simulink model "qless_forgetting_factor_16x16"  (R2021a)
settings: Solver=FixedStepDiscrete  StartTime=0.0  StopTime=stoptime*inf  RelTol=1e-3
InitFcn:
  | qless_init_16chan_fi
undefined symbols (not defined in the file): fc, numArrayElements, physconst, srcAngles, sv, Ts
libraries: hdlsllib x137, commfilt2 x4, commrfcorlib x3, commsync2 x3, commrflib2 x2, commrandsrc3 x2, phasedtxrxlib x2, commdigbbndcpm2 x1, simulink x1, embreciprocals x1, commdigbbndpm3 x1
(part 19 of 22)

== matlab function qless_forgetting_factor_16x16/MVDR_QLess_HDL/Complex Partial-Systolic Matrix Solve Using Q-less QR Decomposition with Forgetting Factor Manually Tiled n=16/Complex Partial-Systolic Q-less QR with Forgetting Factor/Complex Partial-Systolic Q-less QR with Forgetting Factor Manually tiled/Shorten by one3 ==
  data: u input; y output
function y = shorten_by_1(u)
    y = u(2:end);
end

== matlab function qless_forgetting_factor_16x16/MVDR_QLess_HDL/Complex Partial-Systolic Matrix Solve Using Q-less QR Decomposition with Forgetting Factor Manually Tiled n=16/Complex Partial-Systolic Q-less QR with Forgetting Factor/Complex Partial-Systolic Q-less QR with Forgetting Factor Manually tiled/Shorten by one4 ==
  data: u input; y output
function y = shorten_by_1(u)
    y = u(2:end);
end

== matlab function qless_forgetting_factor_16x16/MVDR_QLess_HDL/Complex Partial-Systolic Matrix Solve Using Q-less QR Decomposition with Forgetting Factor Manually Tiled n=16/Complex Partial-Systolic Q-less QR with Forgetting Factor/Complex Partial-Systolic Q-less QR with Forgetting Factor Manually tiled/Shorten by one5 ==
  data: u input; y output
function y = shorten_by_1(u)
    y = u(2:end);
end

== matlab function qless_forgetting_factor_16x16/MVDR_QLess_HDL/Complex Partial-Systolic Matrix Solve Using Q-less QR Decomposition with Forgetting Factor Manually Tiled n=16/Complex Partial-Systolic Q-less QR with Forgetting Factor/Complex Partial-Systolic Q-less QR with Forgetting Factor Manually tiled/Shorten by one6 ==
  data: u input; y output
function y = shorten_by_1(u)
    y = u(2:end);
end

== matlab function qless_forgetting_factor_16x16/MVDR_QLess_HDL/Complex Partial-Systolic Matrix Solve Using Q-less QR Decomposition with Forgetting Factor Manually Tiled n=16/Complex Partial-Systolic Q-less QR with Forgetting Factor/Complex Partial-Systolic Q-less QR with Forgetting Factor Manually tiled/Shorten by one7 ==
  data: u input; y output
function y = shorten_by_1(u)
    y = u(2:end);
end

== matlab function qless_forgetting_factor_16x16/MVDR_QLess_HDL/Complex Partial-Systolic Matrix Solve Using Q-less QR Decomposition with Forgetting Factor Manually Tiled n=16/Complex Partial-Systolic Q-less QR with Forgetting Factor/Complex Partial-Systolic Q-less QR with Forgetting Factor Manually tiled/Shorten by one8 ==
  data: u input; y output
function y = shorten_by_1(u)
    y = u(2:end);
end

== matlab function qless_forgetting_factor_16x16/MVDR_QLess_HDL/Complex Partial-Systolic Matrix Solve Using Q-less QR Decomposition with Forgetting Factor Manually Tiled n=16/Complex Partial-Systolic Q-less QR with Forgetting Factor/Complex Partial-Systolic Q-less QR with Forgetting Factor Manually tiled/Shorten by one10 ==
  data: u input; y output
function y = shorten_by_1(u)
    y = u(2:end);
end

== matlab function qless_forgetting_factor_16x16/MVDR_QLess_HDL/Complex Partial-Systolic Matrix Solve Using Q-less QR Decomposition with Forgetting Factor Manually Tiled n=16/Complex Partial-Systolic Q-less QR with Forgetting Factor/Complex Partial-Systolic Q-less QR with Forgetting Factor Manually tiled/Shorten by one11 ==
  data: u input; y output
function y = shorten_by_1(u)
    y = u(2:end);
end

== matlab function qless_forgetting_factor_16x16/MVDR_QLess_HDL/Complex Partial-Systolic Matrix Solve Using Q-less QR Decomposition with Forgetting Factor Manually Tiled n=16/Complex Partial-Systolic Q-less QR with Forgetting Factor/Complex Partial-Systolic Q-less QR with Forgetting Factor Manually tiled/Shorten by one12 ==
  data: u input; y output
function y = shorten_by_1(u)
    y = u(2:end);
end

== matlab function qless_forgetting_factor_16x16/MVDR_QLess_HDL/Complex Partial-Systolic Matrix Solve Using Q-less QR Decomposition with Forgetting Factor Manually Tiled n=16/Complex Partial-Systolic Q-less QR with Forgetting Factor/Complex Partial-Systolic Q-less QR with Forgetting Factor Manually tiled/Shorten by one13 ==
  data: u input; y output
function y = shorten_by_1(u)
    y = u(2:end);
end

== matlab function qless_forgetting_factor_16x16/MVDR_QLess_HDL/Complex Partial-Systolic Matrix Solve Using Q-less QR Decomposition with Forgetting Factor Manually Tiled n=16/Complex Partial-Systolic Q-less QR with Forgetting Factor/Complex Partial-Systolic Q-less QR with Forgetting Factor Manually tiled/Complex Partial-Systolic Q-less QR Decomposition with Forgetting Factor Section Constant pivot1/Complex Partial-Systolic Q-less QR Row Rotations/Inverse CORDIC Gain1/MATLAB Function ==
  data: u input; y output
function y = inverseCORDICGain(u)
    %inverseCORDICGain Multiply by the inverse of the CORDIC gain constant
    %   Y = inverseCORDICGain(U) multiplies input U by the inverse CORDIC
    %   gain constant.  The data type of output Y is the same as the data
    %   type of input U.  This data type will never overflow because the
    %   inverse CORDIC gain constant quickly converges to around 0.60725 as
    %   a function of the word length of the input.
    F = fixed.fimathLike(u);
    [~, Kn] = fixed.cordicConstants(u);
    y = setfimath(u,F) * Kn;
end

== matlab function qless_forgetting_factor_16x16/MVDR_QLess_HDL/Complex Partial-Systolic Matrix Solve Using Q-less QR Decomposition with Forgetting Factor Manually Tiled n=16/Complex Partial-Systolic Q-less QR with Forgetting Factor/Complex Partial-Systolic Q-less QR with Forgetting Factor Manually tiled/Complex Partial-Systolic Q-less QR Decomposition with Forgetting Factor Section Constant pivot1/Complex Partial-Systolic Q-less QR Row Rotations/Inverse CORDIC Gain4/MATLAB Function ==
  data: u input; y output
function y = inverseCORDICGain(u)
    %inverseCORDICGain Multiply by the inverse of the CORDIC gain constant
    %   Y = inverseCORDICGain(U) multiplies input U by the inverse CORDIC
    %   gain constant.  The data type of output Y is the same as the data
    %   type of input U.  This data type will never overflow because the
    %   inverse CORDIC gain constant quickly converges to around 0.60725 as
    %   a function of the word length of the input.
    F = fixed.fimathLike(u);
    [~, Kn] = fixed.cordicConstants(u);
    y = setfimath(u,F) * Kn;
end

== matlab function qless_forgetting_factor_16x16/MVDR_QLess_HDL/Complex Partial-Systolic Matrix Solve Using Q-less QR Decomposition with Forgetting Factor Manually Tiled n=16/Complex Partial-Systolic Q-less QR with Forgetting Factor/Complex Partial-Systolic Q-less QR with Forgetting Factor Manually tiled/Complex Partial-Systolic Q-less QR Decomposition with Forgetting Factor Section Constant pivot1/Complex Partial-Systolic Q-less QR Row Rotations/Q-less QR Rotate First Element To Real1/Q-less QR Real Row Rotations/Inverse CORDIC Gain/MATLAB Function ==
  data: u input; y output
function y = inverseCORDICGain(u)
    %inverseCORDICGain Multiply by the inverse of the CORDIC gain constant
    %   Y = inverseCORDICGain(U) multiplies input U by the inverse CORDIC
    %   gain constant.  The data type of output Y is the same as the data
    %   type of input U.  This data type will never overflow because the
    %   inverse CORDIC gain constant quickly converges to around 0.60725 as
    %   a function of the word length of the input.
    F = fixed.fimathLike(u);
    [~, Kn] = fixed.cordicConstants(u);
    y = setfimath(u,F) * Kn;
end

== matlab function qless_forgetting_factor_16x16/MVDR_QLess_HDL/Complex Partial-Systolic Matrix Solve Using Q-less QR Decomposition with Forgetting Factor Manually Tiled n=16/Complex Partial-Systolic Q-less QR with Forgetting Factor/Complex Partial-Systolic Q-less QR with Forgetting Factor Manually tiled/Complex Partial-Systolic Q-less QR Decomposition with Forgetting Factor Section Constant pivot1/Complex Partial-Systolic Q-less QR Row Rotations/Q-less QR Rotate First Element To Real1/Q-less QR Real Row Rotations/Inverse CORDIC Gain1/MATLAB Function ==
  data: u input; y output
function y = inverseCORDICGain(u)
    %inverseCORDICGain Multiply by the inverse of the CORDIC gain constant
    %   Y = inverseCORDICGain(U) multiplies input U by the inverse CORDIC
    %   gain constant.  The data type of output Y is the same as the data
    %   type of input U.  This data type will never overflow because the
    %   inverse CORDIC gain constant quickly converges to around 0.60725 as
    %   a function of the word length of the input.
    F = fixed.fimathLike(u);
    [~, Kn] = fixed.cordicConstants(u);
    y = setfimath(u,F) * Kn;
end

== matlab function qless_forgetting_factor_16x16/MVDR_QLess_HDL/Complex Partial-Systolic Matrix Solve Using Q-less QR Decomposition with Forgetting Factor Manually Tiled n=16/Complex Partial-Systolic Q-less QR with Forgetting Factor/Complex Partial-Systolic Q-less QR with Forgetting Factor Manually tiled/Complex Partial-Systolic Q-less QR Decomposition with Forgetting Factor Section Constant pivot1/Complex Partial-Systolic Q-less QR Row Rotations/Q-less QR Rotate First Element To Real1/Q-less QR Real Row Rotations/Q-less QR Real Indexed CORDIC Row Rotation/CORDIC QR Kernel ==
  settings: fimath=hdlfimath
  data: xIn input size=n; yIn input size=n; validIn input; restart input; xOut output size=n; yOut output size=n; n parameter; validOut output boolean; ready output; pivot parameter size=1
function [xOut, yOut, validOut, ready] = cordic_qr_row_rotation(...
                                                xIn, yIn,...
                                                validIn,...
                                                restart,...
                                                n, pivot)... 
    %CORDIC_QR_ROW_ROTATION performs one CORDIC Givens rotation
    % [XOUT, YOUT] = CORDIC_QR_ROW_ROTATION(...
    %                                       XREG,YREG,...
    %                                       XIN,YIN,...
    %                                       PIVOT,...
    %                                       STILLITERATING, ITERATION)
    % performs one iteration of the CORDIC Givens rotation according to
    % the formula below.
    %
    % if real(y(column)) < 0
    %       xOut = x - y/2^iteration
    %       yOut = y + x/2^iteration
    %   else
    %       xOut = x + y/2^iteration
    %       yOut = y - x/2^iteration
    % end
    %
    % The values for X, Y, are taken from XIN, YIN, on the first iteration, 
    % and XREG, YREG on succeeding iterations.
    
    %   Copyright 2018 The MathWorks, Inc.
    
    %#codegen
    
    % Initialize variables to set datatypes
    
    persistent xReg yReg count readyReg
    
    
    
    fixed.emblib.internal.cordicRowRotations.checkValidDatatypes(xIn, yIn,'x','y', 'cordic_qr_row_rotation');
    T = fixed.emblib.internal.cordicRowRotations.getTypesTable(xIn,xIn);
    maxNIters = coder.const(fixed.emblib.internal.cordicRowRotations.getMaxNIters(xIn));
    
    if isempty(xReg)
       xReg = zeros(n,1,'like',T.x);
       yReg = zeros(n,1,'like',T.y);
       count = cast(0,'like',T.count);
       readyReg = true;
    end
    
    if validIn
        iteration = cast(0,'like',count);
        x = cast(xIn,'like',T.x);
        y = cast(yIn,'like',T.y);
    else
        iteration = count;
        x = xReg;
        y = yReg;
    end
    
    
    [xNext, yNext] = cordicQlessQRRowRotation(x, y, iteration, pivot, T);
    incrCounter =  (validIn && readyReg) || (iteration > 0 && iteration < maxNIters);
    if restart || ~incrCounter
        iterationNext = cast(0,'like',T.count);
    else
        iterationNext = cast(iteration + 1,'like',T.count);
    end
    
    if restart || (iteration == maxNIters - 1)
        readyNext = true;
    elseif validIn && ~readyReg
        readyNext = false;
    else
        readyNext = readyReg;
    end
        
        
    % Set the output
    xOut = xNext;
    yOut = yNext;
    if iteration == maxNIters - 1
        validOut = true;
        % Set the registers to zero to prevent overflows being reported on
        % CORDIC iterations over invalid data.
        xReg(:) = 0;
        yReg(:) = 0;
    else
        validOut = false;
        % Still iterating, so update the registers with next values.
        xReg(:) = xNext;
        yReg(:) = yNext;
    end
    ready = readyNext;
    % Update the registers
    count(:) = iterationNext;
    readyReg(:) = readyNext;
    
    
end

function [xOut, yOut] = cordicQlessQRRowRotation(x, y,...
        iteration, pivot, T)
%cordicQlessQRRowRotation One iteration of the Q-less QR CORDIC kernel
%   [XOUT, YOUT] = cordicQlessQRRowRotation(X,Y,...
%                                      ITERATION, PIVOT, T)
%   performs a single CORDIC Givens rotation according to the
%   formula below
%
%   if real(y(pivot)) < 0
%       xOut = x - y/2^iteration
%       yOut = y + x/2^iteration
%   else
%       xOut = x + y/2^iteration
%       yOut = y - x/2^iteration
%   end

    coder.inline('always');
    
    % Initialize output variables
    xOut = cast(x,'like',T.x);
    yOut = cast(y,'like',T.y);
    % Right shift the inputs for CORDIC rotations.
    x1 = zeros(size(x),'like',x);
    y1 = zeros(size(y),'like',y);
    coder.unroll
    for k = pivot:length(x)
        x1(k) = bitsra(x(k), iteration);
        y1(k) = bitsra(y(k), iteration);
    end
    if real(y(pivot)) < 0
        % Counter-clockwise rotation
        coder.unroll
        for k = pivot:length(x)
            xOut(k) = x(k) - y1(k);
            yOut(k) = y(k) + x1(k);
        end
    else
        % Clockwise rotation
        coder.unroll
        for k = pivot:length(x)
            xOut(k) = x(k) + y1(k);
            yOut(k) = y(k) - x1(k);
        end
    end
end

== matlab function qless_forgetting_factor_16x16/MVDR_QLess_HDL/Complex Partial-Systolic Matrix Solve Using Q-less QR Decomposition with Forgetting Factor Manually Tiled n=16/Complex Partial-Systolic Q-less QR with Forgetting Factor/Complex Partial-Systolic Q-less QR with Forgetting Factor Manually tiled/Complex Partial-Systolic Q-less QR Decomposition with Forgetting Factor Section Constant pivot1/Complex Partial-Systolic Q-less QR Row Rotations/Q-less QR Rotate First Element To Real1/Q-less QR Real Row Rotations/Set Element To Zero/Set Element To Zero ==
  settings: fimath=hdlfimath
  data: u input size=[1 n]; y output size=[1 n]; n parameter; pivot parameter size=1
function y = set_element_equal_to_zero(u, n, pivot)
    % SET_ELEMENT_EQUAL_TO_ZERO Zeros an element for a row-vector.
    %   Y = SET_ELEMENT_EQUAL_TO_ZERO(U, PIVOT) sets an element
    %   (specified by PIVOT) of the row-vector U to zero.

    %   Copyright 2018 The MathWorks, Inc.

    %# codegen
    assert(isequal(size(u),[1,n]));
    y = u;
    if pivot > 0 && pivot <= n
        y(pivot) = 0;
    end
end

== matlab function qless_forgetting_factor_16x16/MVDR_QLess_HDL/Complex Partial-Systolic Matrix Solve Using Q-less QR Decomposition with Forgetting Factor Manually Tiled n=16/Complex Partial-Systolic Q-less QR with Forgetting Factor/Complex Partial-Systolic Q-less QR with Forgetting Factor Manually tiled/Shorten by one14 ==
  data: u input; y output
function y = shorten_by_1(u)
    y = u(2:end);
end

== matlab function qless_forgetting_factor_16x16/MVDR_QLess_HDL/Complex Partial-Systolic Matrix Solve Using Q-less QR Decomposition with Forgetting Factor Manually Tiled n=16/Complex Partial-Systolic Q-less QR with Forgetting Factor/Complex Partial-Systolic Q-less QR with Forgetting Factor Manually tiled/Complex Partial-Systolic Q-less QR Decomposition with Forgetting Factor Section Constant pivot1/Complex Partial-Systolic Q-less QR Row Rotations/Set Element To Zero1/Set Element To Zero ==
  settings: fimath=hdlfimath
  data: u input size=[1 n]; y output size=[1 n]; n parameter; pivot parameter size=1
function y = set_element_equal_to_zero(u, n, pivot)
    % SET_ELEMENT_EQUAL_TO_ZERO Zeros an element for a row-vector.
    %   Y = SET_ELEMENT_EQUAL_TO_ZERO(U, PIVOT) sets an element
    %   (specified by PIVOT) of the row-vector U to zero.

    %   Copyright 2018 The MathWorks, Inc.

    %# codegen
    assert(isequal(size(u),[1,n]));
    y = u;
    if pivot > 0 && pivot <= n
        y(pivot) = 0;
    end
end

== matlab function qless_forgetting_factor_16x16/MVDR_QLess_HDL/Complex Partial-Systolic Matrix Solve Using Q-less QR Decomposition with Forgetting Factor Manually Tiled n=16/Complex Partial-Systolic Q-less QR with Forgetting Factor/Complex Partial-Systolic Q-less QR with Forgetting Factor Manually tiled/Complex Partial-Systolic Q-less QR Decomposition with Forgetting Factor Section Constant pivot1/Partial-Systolic Q-less QR with Forgetting Factor Memory Controller/MATLAB Function ==
  data: xIn input; xOut output; aIn input; validIn input size=1; validRowRotationInput input size=1; restart input size=1; yOut output; processRowRotations output size=1; validOut output size=1; ready output size=1; n parameter size=1
function [...
        xOut,...
        yOut,...
        processRowRotations,...
        validOut,...
        ready...
        ] = ...
        partialSystolicQlessQRMemoryControllerForgettingFactorMATLAB(...
        xIn,...
        aIn,...
        validIn,...
        validRowRotationInput,...
        restart, ...
        n)
    
    % Persistent states
    persistent mState
    persistent mRow
    persistent mR
    
    if isempty(mState)
        mState = uint8(0);
        mRow = uint16(1);
        mR = zeros(1,n,'like',aIn);
    end
    
    [...
        xOut,...
        yOut,...
        processRowRotations,...
        validOut,...
        ready,...
        mState,...
        mRow,...
        mR...
        ] = ...
        partialSystolicQlessQRMemoryControllerForgettingFactor(...
        xIn,...
        aIn,...
        validIn,...
        validRowRotationInput,...
        restart, ...
        n,...
        mState,...
        mRow,...
        mR);
end

function [...
        xOut,...
        yOut,...
        processRowRotations,...
        validOut,...
        ready,...
        mState,...
        mRowIndex,...
        mRow...
        ] = ...
        partialSystolicQlessQRMemoryControllerForgettingFactor(...
        xIn,...
        aIn,...
        validIn,...
        validRowRotationInput,...
        restart, ...
        n,...
        mState,...
        mRowIndex,...
        mRow)
    %partialSystolicQlessQRMemoryControllerForgettingFactor
    
    % Copyright 2020 The MathWorks, Inc.
    %#codegen
    
    % State names
    NEWMATRIX = uint8(0);
    GETROW = uint8(1);
    PROCESSPIVOT = uint8(2);
    OUTPUTROW = uint8(3);
    
    % Get states
    state = mState;
    row = mRowIndex;
    
    if restart
        state = NEWMATRIX;
    end
    
    % Default outputs.  States change them as needed.
    xOut = mRow;
    yOut = aIn;
    processRowRotations = false;
    validOut = false;
    ready = false;
    
    switch state
        case NEWMATRIX
            mRow(:) = 0;
            mRowIndex(:) = 1;
            mState(:) = GETROW;
            ready(:) = true;
        case GETROW
            if  validIn
                processRowRotations = true;
                mRowIndex(:) = row + 1;
                mState(:) = PROCESSPIVOT;
            else
                ready = true;
            end
        case PROCESSPIVOT
            if validRowRotationInput
                mRow(:) = xIn;
                if row > n
                    mState(:) = OUTPUTROW;
                else
                    mState(:) = GETROW;
                end
            end
        case OUTPUTROW
            validOut = true;
            mState(:) = GETROW;
    end
end

== matlab function qless_forgetting_factor_16x16/MVDR_QLess_HDL/Complex Partial-Systolic Matrix Solve Using Q-less QR Decomposition with Forgetting Factor Manually Tiled n=16/Complex Partial-Systolic Q-less QR with Forgetting Factor/Complex Partial-Systolic Q-less QR with Forgetting Factor Manually tiled/Shorten by one9 ==
  data: u input; y output
function y = shorten_by_1(u)
    y = u(2:end);
end

== matlab function qless_forgetting_factor_16x16/MVDR_QLess_HDL/Complex Partial-Systolic Matrix Solve Using Q-less QR Decomposition with Forgetting Factor Manually Tiled n=16/Complex Partial-Systolic Q-less QR with Forgetting Factor/Partial-Systolic Q-less QR with Forgetting Factor Output Memory Manager/Partial-Systolic Q-less QR Output Memory Manager1/Partial-Systolic Q-less QR Output State Machine ==
  data: writeEnable output; validIn input; restart input; m parameter size=1; n parameter size=1; validOut output
function [writeEnable,validOut] = qlessqrOutputMATLABFunctionBlock(validIn,restart,m,n)
    coder.internal.assert(m>=n,'fixed:emblib:MustBeTallAndSkinny','A');
    % State names
    NEWMATRIX = uint8(0);
    GETROW = uint8(1);
    persistent mWriteEnable;
    persistent mRowCounter
    persistent mPivot
    persistent mState
    persistent mValidOut
    if isempty(mWriteEnable)
        mWriteEnable = false(1,n);
        mRowCounter = uint32(0);
        mPivot = uint32(1);
        mState = GETROW;
        mValidOut = false;
    end
    writeEnable = mWriteEnable;
    validOut = mValidOut;
    
    state = mState;
    rowCounter = mRowCounter;
    pivot = mPivot;
    mValidOut = false;
    
    if restart
        state = NEWMATRIX;
    end
    mWriteEnable(:) = false;
    switch state
        case NEWMATRIX
            rowCounter(:) = 0;
            pivot(:) = 1;
            state(:) = GETROW;
        case GETROW
            if validIn(pivot)
                mWriteEnable(pivot) = true;
                pivot(:) = pivot + 1;
                if pivot > min(m,n)
                    rowCounter(:) = 1;
                    pivot(:) = 1;
                    mValidOut(:) = true;
                end
            end
        otherwise
    end
    
    mRowCounter(:) = rowCounter;
    mPivot(:) = pivot;
    mState(:) = state;
end

== matlab function qless_forgetting_factor_16x16/MVDR_QLess_HDL/Complex Partial-Systolic Matrix Solve Using Q-less QR Decomposition with Forgetting Factor Manually Tiled n=16/Complex Partial-Systolic Q-less QR with Forgetting Factor/Partial-Systolic Q-less QR with Forgetting Factor Output Memory Manager/Partial-Systolic Q-less QR Output Memory Manager1/Save Matrix Row/Enabled Delay ==
  data: dataIn input; dataOut output; writeEnable input
function dataOut = enabledDelay(dataIn,writeEnable)
    persistent mData
    if isempty(mData)
        mData = zeros(size(dataIn),'like',dataIn);
    end
    dataOut = mData;
    if writeEnable
        mData = dataIn;
    end
end

== matlab function qless_forgetting_factor_16x16/MVDR_QLess_HDL/Complex Partial-Systolic Matrix Solve Using Q-less QR Decomposition with Forgetting Factor Manually Tiled n=16/Complex Q-less QR Forward Backward Substitute/Complex Burst Back Substitute with Matrix Output1/Back substitute logic/Back substitute state machine ==
  settings: fimath=hdlfimath
  data: rowToSubtract1 output size=[1 p]; rowToSubtract2 output size=[1 p]; inverseElement input size=1; inverseShift input size=1; rIn input size=[1 n]; cIn input size=[1 p]; validIn input boolean size=1; start input boolean size=1; restart input boolean size=1; subtractedRow input size=[1 p]; addedRow input size=[1 p]; multipliedRow input size=[1 p]; finalMultipliedRow input size=[1 p]; rowToAdd1 output size=[1 p]; rowToAdd2 output size=[1 p]; rowToMultiply output size=[1 p]; rElement output size=1; finalRowToMultiply output size=[1 p]; reciprocal output size=1; shiftValue output size=1; xMatrix output size=[n p]; ready output boolean size=1; rowReady output boolean size=1; validOut output boolean size=1; n parameter size=1; p parameter size=1
function [rowToSubtract1,...
          rowToSubtract2,...
          rowToAdd1,...
          rowToAdd2,...
          rowToMultiply,...
          rElement,...
          finalRowToMultiply,...
          reciprocal,...
          shiftValue,...
          xMatrix,...
          ready,...
          rowReady,...
          validOut] = backsubStateMachine(inverseElement,...
                                          inverseShift,...
                                          rIn,...
                                          cIn,...
                                          validIn,...
                                          start,...
                                          restart,...
                                          subtractedRow,...
                                          addedRow,...
                                          multipliedRow,...
                                          finalMultipliedRow,...
                                          n,...
                                          p)
%backsubStateMachine Implements a state machine that manages the back
%substitute computation to compute the output matrix.
%
%   See also fixed.internal.matrixsolve.selectDiagonalElement.
%
%   Copyright 2019 The MathWorks, Inc.
%#codegen

%% INPUTS
% 'inverseElement' - The reciprocal of the diagonal element to be used
% later.
%
% 'inverseShift' - The reciprocal of the diagonal element is normalized,
% and needs to be denormalized later to yield the correct value.
%
% 'rIn' - A non-zero row of the R matrix from the QR decomposition.
%
% 'cIn' - A row of the Q'B matrix, where Q is obtained from the QR
% decomposition.
%
% 'validIn' - A boolean signal indicating that the data on the input lines
% is valid.
%
% 'start' - A boolean signal indicating that a new backsubstitute has
% begun; it thus indicates that new data should be expected.
%
% 'restart' - A boolean signal to reset the internal state of the block if
% necessary.
%
% 'subtractedRow' - The result of the subraction of the accumulated
% products of the non-diagonal elements of the supplied 'rIn' with the
% rows of the solution matrix, from 'cIn'.
%
% 'addedRow' - The accumulation of the products of the non-diagonal
% elements of the supplied 'rIn' with the rows of the solution matrix.
%
% 'multipliedRow' - The product of a non-diagonal element of the supplied
% 'rIn' with a row from the solution matrix.
%
% 'finalMultipliedRow' - The multiplication of the 'subractedRow' with the
% 'inverseElement' - after shifting by 'inverseShift', this is thus a row
% of the solution matrix.
%
% 'm' (parameter) - The number of rows in A and B matrices.
%
% 'n' (parameter) - The number of columns in the A matrix (and thus rows
% in the R matrix).
%
% 'p' (parameter) - The number of columns in the B matrix (and thus columns
% in the R matrix).

%% OUTPUTS
% 'rowToSubtract1' - This is essentially 'cIn'; we want to subtract the
% accumulated sum (of the products of the non-diagonal elements of 'rIn'
% with the rows of the solution matrix).
%
% 'rowToSubtract2' - This is the accumulated sum of the products of the
%  non-diagonal elements of 'rIn' with the rows of the solution matrix.
%
% 'rowToAdd1' - This is the accumulated sum, so far, of the products of the
%  non-diagonal elements of 'rIn' with the rows of the solution matrix.
%
% 'rowToAdd2' - This is 'multipliedRow' - the product of a non-diagonal
% element of 'rIn' with a row of the solution matrix.
%
% 'rowToMultiply' - A row of the solution matrix - same as 'previousRow'.

% 'rElement' - A non-diagonal element of the supplied 'rIn', to be used to
% multiply with a row of the solution matrix.
%
% 'finalRowToMultiply' - The result of the subraction of the accumulated
% products of the non-diagonal elements of the supplied 'rIn' with the
% rows of the solution matrix, from 'cIn'.
%
% 'reciprocal' - The reciprocal of the diagonal element - same as
% 'inverseElement'.
%
% 'shiftValue' - An integer value used to denormalize the reciprocal - same
% as 'inverseShift'.
%
% 'xMatrix' - The solution to A\B.
%
% 'ready' - A boolean signal indicating the end of computation for the
% entire backsubstitute; it goes high AFTER all the rows of the solution
% matrix have been streamed out.
%
% 'rowReady' - A boolean signal indicating (to the connected logic in the
% hierarchy) that a row of the solution matrix has been computed, and thus
% to signal that the block is ready to accept new data.
%
% 'validOut' - A boolean signal indicating that the data on the output line
% 'outputRow' is valid.

%% PERSISTENTS
% 'mState' - An integer value to hold the state for this FSM. Full
% specifics are listed as comments for each case for this variable.
%
% 'rowCounter' - An integer tracking the row of the solution matrix we are
% currently working on.
%
% 'iterCounter' - An integer tracking which rows of the solution matrix
% have been fetched from the RAM already.
%
% 'sumOfProducts' - The accumulated sum of the products of the non-diagonal
% elements of the supplied 'rIn' with the rows of the solution matrix.
%
% 'finalRowInternal' - Same as finalMultipliedRow.
%
% 'outputMatrix' - The solution to A\B.
%
% 'ramCycleCounter' - An integer counter to track how many cycles have
% passed by since a row of the solution matrix was requested from the RAM.
%
% 'realComplexCycleCounter' - An integer counter to track how many cycles
% have passed by since a real number was multiplied with a complex vector.
%
% 'complexComplexCycleCounter' - An integer counter to track how many
% cycles have passed by since a complex number was multiplied with a
% complex vector.
persistent mState;
persistent rowCounter;
persistent iterCounter;
persistent sumOfProducts;
persistent finalRowInternal;
persistent outputMatrix;
persistent ramCycleCounter;
persistent realComplexCycleCounter;
persistent complexComplexCycleCounter;

%% Get Constants
isComplex = false;
[defaultState,...
    numRows,...
    numColsB,...
    numRamCycles,...
    numRealComplexMulCycles,...
    numComplexComplexMulCycles] = fixed.internal.matrixsolve.getBacksubStateConstants(n,p,isComplex);

%% MAIN LOOP
if isempty(mState)
    % Default persistents.
    mState                      = defaultState;
    rowCounter                  = numRows;
    iterCounter                 = numRows;
    sumOfProducts               = zeros(1, numColsB, 'like', cIn);
    finalRowInternal            = zeros(1, numColsB, 'like', cIn);
    outputMatrix                = zeros(n, p, 'like', cIn);
    ramCycleCounter             = numRamCycles;
    realComplexCycleCounter     = numRealComplexMulCycles;
    complexComplexCycleCounter  = numComplexComplexMulCycles;
end

% [rowToSubtract1,... % Outputs
%  rowToSubtract2,...
%  rowToAdd1,...
%  rowToAdd2,...
%  rowToMultiply,...
%  rElement,...
%  finalRowToMultiply,...
%  reciprocal,...
%  shiftValue,...
%  xMatrix,...
%  ready,...
%  rowReady,...
%  validOut,...
%  mState,...          % Persistents
%  rowCounter,...
%  iterCounter,...
%  sumOfProducts,...
%  finalRowInternal,...
%  ramCycleCounter,...
%  realComplexCycleCounter,...
%  complexComplexCycleCounter] = ...
%  fixed.internal.matrixsolve.backsubStateMachineStreamOutMatrix( inverseElement,...  % Inputs
%                                                                 inverseShift,...
%                                                                 rIn,...
%                                                                 cIn,...
%                                                                 validIn,...
%                                                                 start,...
%                                                                 subtractedRow,...
%                                                                 addedRow,...
%                                                                 multipliedRow,...
%                                                                 finalMultipliedRow,...
%                                                                 restart,...
%                                                                 numRows,...         % Constants 
%                                                                 numColsB,...                  
%                                                                 numRamCycles,...                
%                                                                 numRealComplexMulCycles,...
%                                                                 numComplexComplexMulCycles,...
%                                                                 mState,...          % Persistents
%                                                                 rowCounter,...
%                                                                 iterCounter,...
%                                                                 sumOfProducts,...
%                                                                 finalRowInternal,...
%                                                                 outputMatrix,...
%                                                                 ramCycleCounter,...
%                                                                 realComplexCycleCounter,...
%                                                                 complexComplexCycleCounter);

% Describe all possible states.
numStates                   = coder.const(uint8(10));
statesNT                    = numerictype(0, nextpow2(numStates), 0);
defaultState                = fi(0, statesNT);
waitForValidInState         = fi(1, statesNT);
waitForFinalAnswerState     = fi(2, statesNT);
waitForMultiplicationState  = fi(3, statesNT);
waitForAdditionState        = fi(4, statesNT);
waitForSubtractionState     = fi(7, statesNT);

% MAIN LOOP
% NOTE: 'cIn' has the same type as 'previousRow', so they can be used
% interchangeably.

% Default outputs.
rowToSubtract1              = cIn;
rowToSubtract2              = zeros(1, numColsB, 'like', cIn);
rowToAdd1                   = zeros(1, numColsB, 'like', cIn);
rowToAdd2                   = zeros(1, numColsB, 'like', cIn);
rowToMultiply               = zeros(1, numColsB, 'like', cIn);
rElement                    = cast(1, 'like', rIn);
finalRowToMultiply          = cIn;
reciprocal                  = inverseElement;
shiftValue                  = int32(0);
xMatrix                     = zeros(numRows, numColsB, 'like', cIn);
ready                       = false;
rowReady                    = false;
validOut                    = false;

if restart
     % Default persistents.
     isComplex = coder.const(any(~isreal(cIn)));
    [mState,...
    rowCounter,...
    iterCounter,...
    sumOfProducts,...
    finalRowInternal,...
    ramCycleCounter,...
    realComplexCycleCounter,...
    complexComplexCycleCounter] = fixed.internal.matrixsolve.setDefaultPersistentVars(numRows, numColsB, isComplex, cIn);
    outputMatrix = zeros(numRows, numColsB, 'like', cIn);
else
    switch mState
        % STATE 0 - Default case - we end up here at the beginning and
        % the end of each computation, never in between. Wait for 'start'
        % and validIn to go high.
        case defaultState
            % If both 'start' and 'validIn' are high, go to state 2
            % directly and wait for 'finalMultipliedRow'.
            if start && validIn
                rowCounter = numRows;
                mState     = waitForFinalAnswerState;
                % Otherwise, go to state 1 and wait for 'validIn'.
            elseif start
                mState     = waitForValidInState;
                ready      = true;
                % Otherwise, stay here and wait for 'start'/'validIn'.
            else
                mState     = defaultState;
                ready      = true;
            end
            
            % STATE 1 - Wait for 'validIn', but also move to other states
            % depending on some internal variables.
        case waitForValidInState
            % How many iterations do we need?
            iterCounter = numRows;
            
            % Are we done already? Check 'rowCounter' to find out; if yes,
            % stream out the matrix and move to default state.
            if isequal(rowCounter, 0)
                mState          = defaultState;
                ready           = true;
                validOut        = true;
                xMatrix         = outputMatrix;
                rowCounter(:)   = numRows;
                % If this is the first row (from the bottom), then move to
                % state 2 to wait for the final row.
            elseif validIn && isequal(rowCounter, numRows)
                mState          = waitForFinalAnswerState;
                % If not, then multiply previous row with last element of
                % 'rIn'. Then go to state 3, which is the dedicated
                % multiplication state
            elseif validIn
                rowToMultiply   = outputMatrix(numRows, :);
                rElement        = rIn(numRows);
                mState          = waitForMultiplicationState;
            else
                mState(:)       = waitForValidInState;
            end
            
            % STATE 2 - Wait for 'finalMultipliedRow'.
        case waitForFinalAnswerState
            shiftValue(:)                   = inverseShift;
            finalRowToMultiply              = finalRowInternal;
            % If we get the data on this cycle...
            if isequal(realComplexCycleCounter, 1)
                outputMatrix(rowCounter, :) = finalMultipliedRow;
                % Give values to persistent variables for the next cycle, and set
                % 'rowReady' to high.
                rowReady                    = true;
                mState                      = waitForValidInState;
                realComplexCycleCounter     = numRealComplexMulCycles;
                rowCounter(:)               = rowCounter - 1;
                % ...otherwise, wait here.
            else
                realComplexCycleCounter(:)  = realComplexCycleCounter - 1;
            end
            
            % STATE 3 - Wait for 'multipliedRow'.
        case waitForMultiplicationState
            shiftValue(:)                     = 0;
            % If we get the data on this cycle...
            if isequal(complexComplexCycleCounter, 1)
                % Add the new 'multipliedRow' to the accumulated sum of
                % products so far, and move to state 4.
                rowToAdd1                     = sumOfProducts;
                rowToAdd2                     = multipliedRow;
                mState                        = waitForAdditionState;
                iterCounter(:)                = iterCounter - 1;
                complexComplexCycleCounter    = numComplexComplexMulCycles;
                % ...otherwise, wait here.
            else
                complexComplexCycleCounter(:) = complexComplexCycleCounter - 1;
            end
            
            % STATE 4 - Wait for 'addedRow'. Since addition only takes a single
            % cycle, when we get here we should already have the addition.
        case waitForAdditionState
            sumOfProducts       = addedRow;
            % Now do we go back and do more multiplications, or do we go to
            % subtract the accumulated sum from 'cIn'?
            if isequal(iterCounter, rowCounter)
                rowToSubtract1  = cIn;
                rowToSubtract2  = addedRow;
                mState          = waitForSubtractionState;
            else
                % If iterations are left, fetch more data from the RAM.
                rowToMultiply   = outputMatrix(iterCounter, :);
                rElement        = rIn(iterCounter);
                mState          = waitForMultiplicationState;
            end
            
            % STATE 7 - Wait for 'subtractedRow'. Since subtraction only takes
            % a single cycle, when we get here we should already have the
            % subtraction. Then move to state 2 to get 'finalMultipliedRow'.
        case waitForSubtractionState
            reciprocal          = inverseElement;
            finalRowToMultiply  = subtractedRow;
            mState              = waitForFinalAnswerState;
            sumOfProducts       = zeros(1, numColsB, 'like', cIn);
            finalRowInternal    = subtractedRow;
            
            % Catch all other states and go to the default state. Also set all
            % persistent variables to their default values.
        otherwise
            mState                      = defaultState;
            rowCounter                  = numRows;
            iterCounter                 = numRows;
            sumOfProducts               = zeros(1, numColsB, 'like', cIn);
            finalRowInternal            = zeros(1, numColsB, 'like', cIn);
            ramCycleCounter             = numRamCycles;
            realComplexCycleCounter     = numRealComplexMulCycles;
            complexComplexCycleCounter  = numComplexComplexMulCycles;
    end
end


end

== matlab function qless_forgetting_factor_16x16/MVDR_QLess_HDL/Complex Partial-Systolic Matrix Solve Using Q-less QR Decomposition with Forgetting Factor Manually Tiled n=16/Complex Q-less QR Forward Backward Substitute/Complex Burst Back Substitute with Matrix Output1/Back substitute logic/Variable shift/MATLAB Function ==
  settings: fimath=hdlfimath
  data: x input size=[1 p]; y output size=[1 p]; shiftValue input
function y = fcn(x,shiftValue)
    if isfi(x) && isscaledtype(x)
        y = bitshift(x, shiftValue);
    else
        y = cast(double(x)* 2.^double(shiftValue),'like',x);
    end
end

== matlab function qless_forgetting_factor_16x16/MVDR_QLess_HDL/Complex Partial-Systolic Matrix Solve Using Q-less QR Decomposition with Forgetting Factor Manually Tiled n=16/Complex Q-less QR Forward Backward Substitute/Complex Burst Back Substitute with Matrix Output1/Cast to Union of Types ==
  settings: fimath=hdlfimath
  data: Xref input; Cout output; Cin input
function Cout = castToUnionType(Xref,Cin)
    %castToUnionType Cast second input to union of the two types
    T = fixed.internal.type.unionPrototype(Cin,Xref,...
        'RoundingMethod','Floor',...
        'OverflowAction','Wrap');
    Cout = cast(Cin,'like',T);
end

== matlab function qless_forgetting_factor_16x16/MVDR_QLess_HDL/Complex Partial-Systolic Matrix Solve Using Q-less QR Decomposition with Forgetting Factor Manually Tiled n=16/Complex Q-less QR Forward Backward Substitute/Complex Burst Back Substitute with Matrix Output1/Reciprocal of the diagonal element/Positive Normalized Reciprocal HDL Optimized/Positive Real CORDIC Reciprocal Kernel HDL Optimized/positiveNormalizedCORDICReciprocal ==
  settings: fimath=hdlfimath
  data: x input; t_in input; y output; t output; validIn input; validOut output
function [y, t, validOut] = positiveNormalizedCORDICReciprocal(x, t_in, validIn)
%positiveNormalizedCORDICReciprocal Positive normalized reciprocal
%   [y, t, validOut] = positiveNormalizedCORDICReciprocal(x, t_in, validIn)
%   produces y = 1/x when 1 <= x < 2, and t = t_in.
%
%   When x = 0 and x is fixed-point or scaled-double, then y = 2 - eps(y).
%
%   When x = 0 and x is a floating-point type, then y = inf.
%
%   If x is fixed-point, then y is fixed-point with
%   numerictype(1, x.WordLength, x.WordLength - 2).
%
%   If x is floating-point, then y is floating-point of the same type.
%
%   References:
%
%   [1] Jack E. Volder, "The CORDIC Trigonometric Computing Technique," IRE
%       Transactions on Electronic Computers, Volume EC-8, September 1959,
%       pp. 330-334.
%
%   [2] J.S. Walther, "A Unified Algorithm for Elementary Functions,"
%       Conference Proceedings, Spring Joint Computer Conference, May 1971,
%       pp. 379-385.
%
%   See also fixed.internal.reciprocal.cordicReciprocalKernel.

%   Copyright 2019 The MathWorks, Inc.
%#codegen
    fixed.internal.reciprocal.validateReciprocalInputs(x, validIn);
    if isfi(x) && isscaledtype(x)
        % CORDIC reciprocal for fixed-point and scaled-double types
        [y,t,validOut] = fixedpointReciprocal(x,t_in,validIn);
    else
        % y = 1/x for builtin types.
        y = 1./x;
        t = t_in;
        validOut = validIn;
    end
end

function [reciprocal, t, validOut] = fixedpointReciprocal(xIn,t_in, validIn)
%fixedpointReciprocal Fixed-point reciprocal
%   [reciprocal, t, validOut] = fixedpointReciprocal(xIn, t_in, validIn)
%   Given real scalar xIn such that 1 <= xIn < 2 this function produces
%   reciprocal such that
%
%      reciprocal = 1/xIn.
%
%   and reciprocal is in the range 0.5 < reciprocal <= 1.
%
%   When xIn = 0, then y = 2 - eps(y).
%
%   The input is only valid when validIn = true.  The output is only
%   valid when validOut = true.
%
%   The output t is identical to t_in, synchronized by validIn/validOut.
    [T,NumberOfCordicIterations] = fixed.internal.reciprocal.positiveReciprocalTypes(xIn);
    % Register variables for the CORDIC Reciprocal Kernel
    persistent xReg yReg zReg validReg tReg
    if isempty(xReg)
        xReg = zeros(NumberOfCordicIterations+2,1,'like',T.x);
        yReg = zeros(NumberOfCordicIterations+2,1,'like',T.x);
        zReg = zeros(NumberOfCordicIterations+2,1,'like',T.x);
        validReg = zeros(NumberOfCordicIterations+2,1,'like',validIn);
        tReg = zeros(NumberOfCordicIterations+2,1,'like',t_in);
    end
    % CORDIC Reciprocal Kernel
    [reciprocal,t,validOut,...
        xReg,yReg,zReg,validReg,tReg... % Persistent variables
        ] = fixed.internal.reciprocal.cordicReciprocalKernel(xIn,t_in,validIn,...
        xReg,yReg,zReg,validReg,tReg... % Persistent variables
        );
end

== matlab function qless_forgetting_factor_16x16/MVDR MATLAB/MATLAB Function ==
  data: X input; Y output; sv input
function Y = mvdr_beamform(X,sv)

% form covariance matrix
Ecx = X.'*conj(X);

% compute weight vector
wp = Ecx\sv;

% normalize response
w = wp/(sv'*wp);

% form output beam
Y = X*conj(w);

end

== matlab function qless_forgetting_factor_16x16/MVDR_QLess_HDL/Complex Partial-Systolic Matrix Solve Using Q-less QR Decomposition with Forgetting Factor Manually Tiled n=16/Complex Q-less QR Forward Backward Substitute/Complex Burst Back Substitute with Matrix Output1/Reciprocal of the diagonal element/Positive Normalized Reciprocal HDL Optimized/Positive Real Normalizer HDL Optimized/positiveRealNormalizer ==
  settings: fimath=hdlfimath
  data: u input; x output; validIn input; e output; validOut output
function [x, e, validOut] = positiveRealNormalizer(u, validIn)
%positiveRealNormalizer  Positive real normalizer
%   [x, e, validOut] = positiveRealNormalizer(u, validIn) produces
%   x such that 1 <= x < 2 and e such that x = (2^e)*u when u > 0.
%
%   When u = 0 and u is fixed-point or scaled-double, then x = 0 and
%   e = (2^nextpow2(x.WordLength)) - x.WordLength - x.FractionLength.
%
%   When u = 0 and u is floating-point, then x = 0 and e = 1.
%
%   See also fixed.internal.reciprocal.normalizePositiveFixedPoint,
%   fixed.internal.reciprocal.normalizePositiveFloatOrScaledDouble.

%   Copyright 2019 The MathWorks, Inc.
%#codegen

% This function only works on scalars.
% Only operate on the real part
    fixed.internal.reciprocal.validateNormalizerInputs(u, validIn);
    % Normalize in unsigned type.
    [x_normalized, n_normalized, validOut] = normalize(real(u), validIn);
    % Cast the output to signed if the input was signed.
    x = fixed.internal.reciprocal.castToInputSignedness(x_normalized,u);
    % Convert the normalized shift value based on the data type of the
    % input U so that the output of the normalizer X is in real-world
    % scale and X = (2^N)*U.
    e = fi(int32(0));
    e(:) = fixed.internal.reciprocal.normalizedShiftToRealWorldValueShift(n_normalized,u);
end

function [x_normalized, e_normalized, validOut] = normalize(u, validIn)
    if isfi(u) && isfixed(u)
        % Normalize fixed-point values
        [x_normalized, e_normalized,validOut] = normalizeFixedpoint(u, validIn);
    else
        % Normalize floating-point or scaled-double
        [x_normalized, e_normalized, validOut] = fixed.internal.reciprocal.normalizePositiveFloatOrScaledDouble(u, validIn);
    end
end

function [u_normalized, e_normalized,validOut] = normalizeFixedpoint(u, validIn)
% Normalize fixed-point values.
    persistent validReg
    persistent tReg
    persistent xReg
    % For fixed-point types, the normalization uses a binary search of
    % length log2 of the word length of the input.
    number_of_stages = coder.const(nextpow2(u.WordLength));

    if isempty(validReg)
        validReg = false(number_of_stages+1,1);
        tReg = zeros(number_of_stages+1,1,'like',fi(0,0,max(number_of_stages,1),0));
        xReg = zeros(number_of_stages+1,1,'like',fi([],0,u.WordLength,0));
    end

    [u_normalized, e_normalized,validOut,...
        validReg, tReg,xReg...  % Persistent
        ] = fixed.internal.reciprocal.normalizePositiveFixedPoint(u, validIn, number_of_stages, ...
        validReg, tReg,xReg...  % Persistent
        );
end
